simulink model "sinlgeTetherNGreater2_th"  (R2018b)
settings: Solver=ode15s  StartTime=0.0  StopTime=sim_time  FixedStep=dt  MaxStep=dt  RelTol=1e-3
values from neighbouring files (symbols this model uses):
  amp = 10    [singleTether_ts.m]
  flow = [1 0 0]'    [singleTether_ts.m]
  g = 9.81    [singleTether_ts.m]
  L = 100    [singleTether_ts.m]
  N = sim_param.N    [singleTether_ts.m]
  omega = 1    [singleTether_ts.m]
  R1_o = [0 0 0]'    [singleTether_ts.m]
  V1_o = [0 0 0]'    [singleTether_ts.m]
libraries: singleTetherNGreater2_cl x1
settings Model: Creator=asiddiq2  LastModifiedBy=asiddiq2

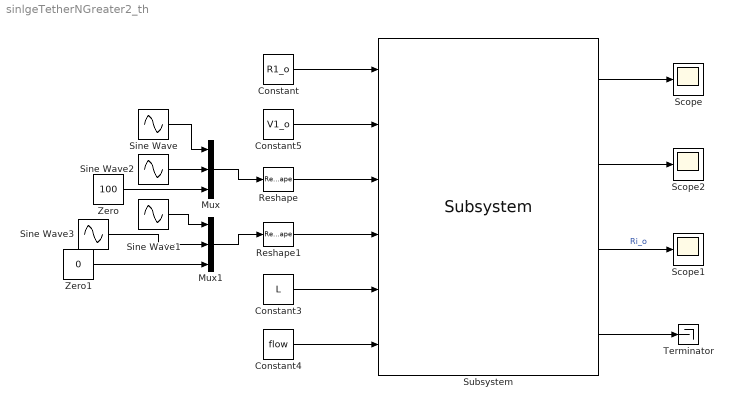
== system sinlgeTetherNGreater2_th ==
  Constant : Constant  Value=R1_o
  Constant3 : Constant  Value=L
  Constant4 : Constant  Value=flow
  Constant5 : Constant  Value=V1_o
  Mux : Mux  Inputs=3
  Mux1 : Mux  Inputs=3
  Reshape : Reshape  OutputDimensionality=Column vector (2-D)
  Reshape1 : Reshape  OutputDimensionality=Column vector (2-D)
  Scope : Scope
  Scope1 : Scope
  Scope2 : Scope
  Sine Wave : Sin  Amplitude=amp  Frequency=omega  Phase=pi/2  SampleTime=0
  Sine Wave1 : Sin  Amplitude=-amp*omega  Frequency=omega  SampleTime=0
  Sine Wave2 : Sin  Amplitude=amp  Frequency=omega  SampleTime=0
  Sine Wave3 : Sin  Amplitude=amp*omega  Frequency=omega  Phase=pi/2  SampleTime=0
  Subsystem : singleTetherNGreater2_cl/Subsystem  N=N  dia_t=dia_t  E=E  rho_tether=rho_tether  Cd=Cd  zeta=zeta  rho=rho_fluid  g=g  mass=mass  ini_Rn_o=Rn_o  ini_R1_o=R1_o
  Terminator : Terminator
  Zero : Constant  Value=100  OutDataTypeStr=Inherit: Inherit via back propagation
  Zero1 : Constant  Value=0  OutDataTypeStr=Inherit: Inherit via back propagation
  wires:
  Constant3/1 -> Subsystem/5
  Constant4/1 -> Subsystem/6
  Constant5/1 -> Subsystem/2
  Subsystem/1 -> Scope/1
  Mux/1 -> Reshape/1
  Reshape/1 -> Subsystem/3
  Sine Wave/1 -> Mux/1
  Constant/1 -> Subsystem/1
  Reshape1/1 -> Subsystem/4
  Sine Wave1/1 -> Mux1/1
  Mux1/1 -> Reshape1/1
  Zero/1 -> Mux/3
  Sine Wave2/1 -> Mux/2
  Zero1/1 -> Mux1/3
  Sine Wave3/1 -> Mux1/2
  Subsystem/3 -> Scope1/1  "Ri_o"
  Subsystem/4 -> Terminator/1
  Subsystem/2 -> Scope2/1
